simulink model "Parameter_estimation1"  (R2025b)
settings: Solver=VariableStepAuto  StartTime=0.0  StopTime=206057  FixedStep=1
libraries: fl_lib x15, nesl_utility x15, batt_lib x7, ee_lib x3
settings Model: Creator=faxio  LastModifiedBy=faxio

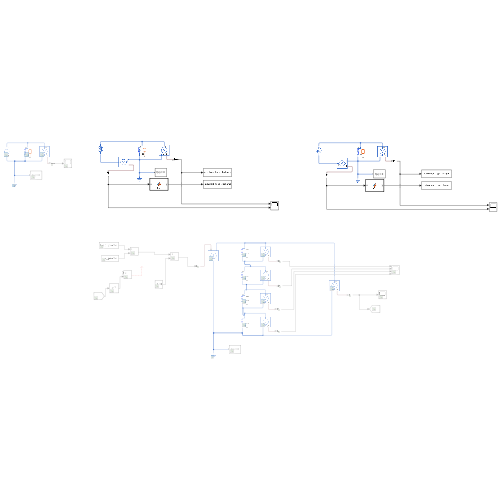
[thumbnail: Simulink's stored preview of the top-level diagram]
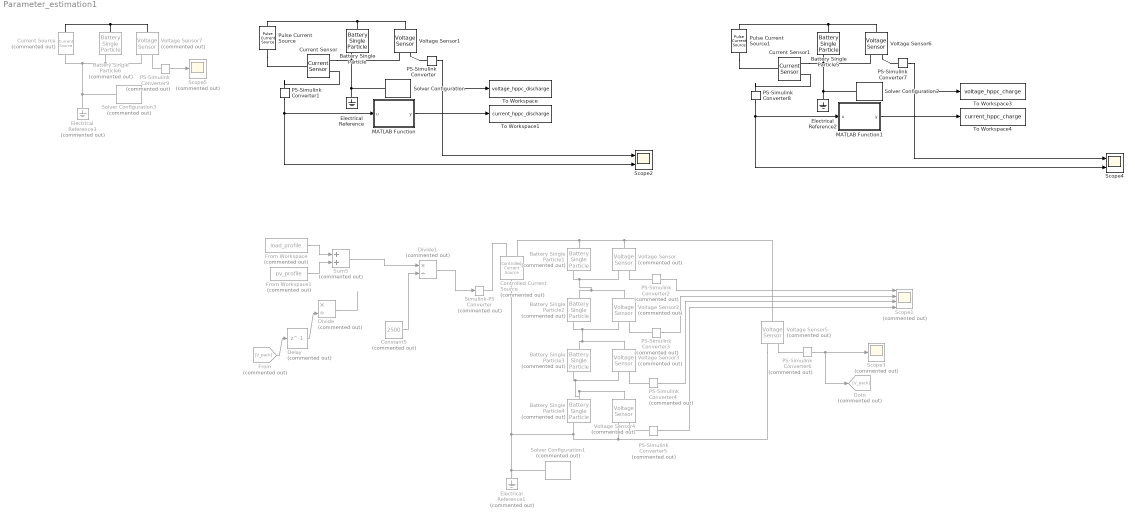
== system Parameter_estimation1 ==
  Battery Single Particle : batt_lib/Cells/Electrochemical/Battery Single Particle  ExtrapolationMethod=simscape.enum.extrapolation.nearest  ThicknessAnode=3.4E-5 m  ElectrolyteLayerCountAnode=10  ThicknessSeparator=2.5E-5 m  ElectrolyteLayerCountSeparator=5  ThicknessCathode=8E-5 m  ElectrolyteLayerCountCathode=10  ElectrodePlateArea=1.8E-1 m^2  ParticleRadiusAnode=5E-6 m  ShellCountAnode=10  ParticleRadiusCathode=5E-8 m  ShellCountCathode=10  ActiveMaterialVolumeFractionAnode=0.58  ActiveMaterialVolumeFractionCathode=0.374  StoichiometryBreakpointsSpecification=simscape.battery.enum.cells.electrochemical.StoichiometryBreakpointsSpecification.normalized  NormalizedStoichiometryBreakpoints=linspace(0.025, 0.975, 39)  OpenCircuitPotentialAnode=[.435; .325; .259; .221; .204; .194; .179; .166; .155; .145; .137; .131; .128; .127; .126; .125; .124; .123; .122; .121; .118; .117; .112; .109; .105; .1; .098; .095; .094; .093; .091; .09; .089; .088; .087; .086; .085; .084; .083] V  OpenCircuitPotentialCathode=[3.598; 3.53; 3.494; 3.474; 3.46; 3.455; 3.454; 3.453; 3.4528; 3.4526; 3.4524; 3.452; 3.4518; 3.4516; 3.4514; 3.4512; 3.451; 3.4508; 3.4506; 3.4503; 3.45; 3.4498; 3.4495; 3.4493; 3.449; 3.4488; 3.4486; 3.4484; 3.4482; 3.4479; 3.4477; 3.4475; 3.4473; 3.447; 3.4468; 3.4466; 3.4464; 3.4462; 3.4458] V  AbsoluteStoichiometryBreakpointsAnode=linspace(0.025, 0.975, 39)  OpenCircuitPotentialAbsoluteAnode=[.484; .335; .253; .209; .2; .181; .165; .151; .139; .131; .128; .125; .124; .124; .123; .122; .119; .117; .111; .108; .101; .098; .095; .093; .092; .088; .088; .088; .088; .087; .087; .087; .085; .082; .079; .071; .064; .049; .026] V  AbsoluteStoichiometryBreakpointsCathode=linspace(0.025, 0.975, 39)  OpenCircuitPotentialAbsoluteCathode=[3.81; 3.608; 3.512; 3.478; 3.459; 3.453; 3.45257; 3.45214; 3.45171; 3.45128; 3.45085; 3.45042; 3.44999; 3.44956; 3.44913; 3.4487; 3.44827; 3.44784; 3.44741; 3.44698; 3.44655; 3.44612; 3.44569; 3.44526; 3.44483; 3.4444; 3.44397; 3.44354; 3.44311; 3.44268; 3.44225; 3.44182; 3.44139; 3.44096; 3.44053; 3.44; 3.412; 3.304; 2.968] V  MaximumConcentrationAnode=30555 mol/m^3  MaximumStoichiometryAnode=0.811  MinimumStoichiometryAnode=0.0132  MaximumConcentrationCathode=22806 mol/m^3  MaximumStoichiometryCathode=0.74  MinimumStoichiometryCathode=0.035  ActiveMaterialDiffusionCoefficientAnode=3E-15 m^2/s  ActiveMaterialDiffusionCoefficientCathode=5.9E-20 m^2/s  ConductivityAnode=100 S/m  ConductivityCathode=0.5 S/m  CurrentCollectorResistance=0 Ohm  ElectrolyteVolumeFractionAnode=0.3874  ElectrolyteVolumeFractionSeparator=0.45  ElectrolyteVolumeFractionCathode=0.5725  ElectrolyteConductivity=0.29 S/m  BruggemanExponentAnode=1.5  BruggemanExponentSeparator=1.5  BruggemanExponentCathode=1.5  TransferenceNumber=0.363  ElectrolyteDiffusionCoefficient=2E-10 m^2/s  ChargeTransferRateAnode=8.8E-11 m^(5/2)/(mol^(1/2)*s)  ChargeTransferRateCathode=2.8E-13 m^(5/2)/(mol^(1/2)*s)  BatteryThermalMass=77 J/K  ArrheniusReferenceTemperature=298.15 K  ActiveMaterialDiffusionActivationEnergyAnode=39000 J/mol  ActiveMaterialDiffusionActivationEnergyCathode=35000 J/mol  ElectrolyteDiffusionActivationEnergy=26600 J/mol  ConductivityActivationEnergyAnode=3000 J/mol  ConductivityActivationEnergyCathode=3000 J/mol  ElectrolyteConductivityActivationEnergy=11000 J/mol  ChargeTransferActivationEnergyAnode=13000 J/mol  ChargeTransferActivationEnergyCathode=20000 J/mol  batteryCurrent_specify=off  batteryCurrent_priority=None  batteryCurrent=0 A  batteryCurrent_nominal_specify=off  batteryCurrent_nominal_value=1  batteryCurrent_nominal_unit=A  batteryVoltage_specify=off  batteryVoltage_priority=None  batteryVoltage=0 V  batteryVoltage_nominal_specify=off  batteryVoltage_nominal_value=1  batteryVoltage_nominal_unit=V  averageElectrolyteConcentration_specify=off  averageElectrolyteConcentration_priority=High  averageElectrolyteConcentration=1200 mol/m^3  averageElectrolyteConcentration_nominal_specify=off  averageElectrolyteConcentration_nominal_value=1  averageElectrolyteConcentration_nominal_unit=mol/m^3  stateOfCharge_specify=on  stateOfCharge_priority=High  stateOfCharge=1  stateOfCharge_nominal_specify=off  stateOfCharge_nominal_value=1  stateOfCharge_nominal_unit=1  batteryTemperature_specify=off  batteryTemperature_priority=High  batteryTemperature=298.15 K  batteryTemperature_nominal_specify=off  batteryTemperature_nominal_value=1  batteryTemperature_nominal_unit=K  power_dissipated_specify=off  power_dissipated_priority=None  power_dissipated=0 W  power_dissipated_nominal_specify=off  power_dissipated_nominal_value=1  power_dissipated_nominal_unit=W  heatGenerationRate_specify=off  heatGenerationRate_priority=None  heatGenerationRate=0 W  heatGenerationRate_nominal_specify=off  heatGenerationRate_nominal_value=1  heatGenerationRate_nominal_unit=W
      settings: InternalSimscapePortConfiguration="{\"Bottom\":[],\"Left\":[{\"id\":\"p\",\"label\":\"+\",\"type\":\"foundation.electrical.electrical\"}],\"Right\":[{\"id\":\"n\",\"label\":\"-\",\"type\":\"foundation.electrical.electrical\"},{\"id\":\"H\",\"label\":\"H\",\"type\":\"foundation.thermal.thermal\"}],\"Top\":[]}"
  Battery Single Particle{1..4,6} (5 alike) : batt_lib/Cells/Electrochemical/Battery Single Particle  Commented=on  ExtrapolationMethod=simscape.enum.extrapolation.nearest  ThicknessAnode=3.4E-5 m  ElectrolyteLayerCountAnode=10  ThicknessSeparator=2.5E-5 m  ElectrolyteLayerCountSeparator=5  ThicknessCathode=8E-5 m  ElectrolyteLayerCountCathode=10  ElectrodePlateArea=1.8E-1 m^2  ParticleRadiusAnode=5E-6 m  ShellCountAnode=10  ParticleRadiusCathode=5E-8 m  ShellCountCathode=10  ActiveMaterialVolumeFractionAnode=0.58  ActiveMaterialVolumeFractionCathode=0.374  StoichiometryBreakpointsSpecification=simscape.battery.enum.cells.electrochemical.StoichiometryBreakpointsSpecification.normalized  NormalizedStoichiometryBreakpoints=linspace(0.025, 0.975, 39)  OpenCircuitPotentialAnode=[.435; .325; .259; .221; .204; .194; .179; .166; .155; .145; .137; .131; .128; .127; .126; .125; .124; .123; .122; .121; .118; .117; .112; .109; .105; .1; .098; .095; .094; .093; .091; .09; .089; .088; .087; .086; .085; .084; .083] V  OpenCircuitPotentialCathode=[3.598; 3.53; 3.494; 3.474; 3.46; 3.455; 3.454; 3.453; 3.4528; 3.4526; 3.4524; 3.452; 3.4518; 3.4516; 3.4514; 3.4512; 3.451; 3.4508; 3.4506; 3.4503; 3.45; 3.4498; 3.4495; 3.4493; 3.449; 3.4488; 3.4486; 3.4484; 3.4482; 3.4479; 3.4477; 3.4475; 3.4473; 3.447; 3.4468; 3.4466; 3.4464; 3.4462; 3.4458] V  AbsoluteStoichiometryBreakpointsAnode=linspace(0.025, 0.975, 39)  OpenCircuitPotentialAbsoluteAnode=[.484; .335; .253; .209; .2; .181; .165; .151; .139; .131; .128; .125; .124; .124; .123; .122; .119; .117; .111; .108; .101; .098; .095; .093; .092; .088; .088; .088; .088; .087; .087; .087; .085; .082; .079; .071; .064; .049; .026] V  AbsoluteStoichiometryBreakpointsCathode=linspace(0.025, 0.975, 39)  OpenCircuitPotentialAbsoluteCathode=[3.81; 3.608; 3.512; 3.478; 3.459; 3.453; 3.45257; 3.45214; 3.45171; 3.45128; 3.45085; 3.45042; 3.44999; 3.44956; 3.44913; 3.4487; 3.44827; 3.44784; 3.44741; 3.44698; 3.44655; 3.44612; 3.44569; 3.44526; 3.44483; 3.4444; 3.44397; 3.44354; 3.44311; 3.44268; 3.44225; 3.44182; 3.44139; 3.44096; 3.44053; 3.44; 3.412; 3.304; 2.968] V  MaximumConcentrationAnode=30555 mol/m^3  MaximumStoichiometryAnode=0.811  MinimumStoichiometryAnode=0.0132  MaximumConcentrationCathode=22806 mol/m^3  MaximumStoichiometryCathode=0.74  MinimumStoichiometryCathode=0.035  ActiveMaterialDiffusionCoefficientAnode=3E-15 m^2/s  ActiveMaterialDiffusionCoefficientCathode=5.9E-20 m^2/s  ConductivityAnode=100 S/m  ConductivityCathode=0.5 S/m  CurrentCollectorResistance=0 Ohm  ElectrolyteVolumeFractionAnode=0.3874  ElectrolyteVolumeFractionSeparator=0.45  ElectrolyteVolumeFractionCathode=0.5725  ElectrolyteConductivity=0.29 S/m  BruggemanExponentAnode=1.5  BruggemanExponentSeparator=1.5  BruggemanExponentCathode=1.5  TransferenceNumber=0.363  ElectrolyteDiffusionCoefficient=2E-10 m^2/s  ChargeTransferRateAnode=8.8E-11 m^(5/2)/(mol^(1/2)*s)  ChargeTransferRateCathode=2.8E-13 m^(5/2)/(mol^(1/2)*s)  BatteryThermalMass=77 J/K  ArrheniusReferenceTemperature=298.15 K  ActiveMaterialDiffusionActivationEnergyAnode=39000 J/mol  ActiveMaterialDiffusionActivationEnergyCathode=35000 J/mol  ElectrolyteDiffusionActivationEnergy=26600 J/mol  ConductivityActivationEnergyAnode=3000 J/mol  ConductivityActivationEnergyCathode=3000 J/mol  ElectrolyteConductivityActivationEnergy=11000 J/mol  ChargeTransferActivationEnergyAnode=13000 J/mol  ChargeTransferActivationEnergyCathode=20000 J/mol  batteryCurrent_specify=off  batteryCurrent_priority=None  batteryCurrent=0 A  batteryCurrent_nominal_specify=off  batteryCurrent_nominal_value=1  batteryCurrent_nominal_unit=A  batteryVoltage_specify=off  batteryVoltage_priority=None  batteryVoltage=0 V  batteryVoltage_nominal_specify=off  batteryVoltage_nominal_value=1  batteryVoltage_nominal_unit=V  averageElectrolyteConcentration_specify=off  averageElectrolyteConcentration_priority=High  averageElectrolyteConcentration=1200 mol/m^3  averageElectrolyteConcentration_nominal_specify=off  averageElectrolyteConcentration_nominal_value=1  averageElectrolyteConcentration_nominal_unit=mol/m^3  stateOfCharge_specify=on  stateOfCharge_priority=High  stateOfCharge=1  stateOfCharge_nominal_specify=off  stateOfCharge_nominal_value=1  stateOfCharge_nominal_unit=1  batteryTemperature_specify=off  batteryTemperature_priority=High  batteryTemperature=298.15 K  batteryTemperature_nominal_specify=off  batteryTemperature_nominal_value=1  batteryTemperature_nominal_unit=K  power_dissipated_specify=off  power_dissipated_priority=None  power_dissipated=0 W  power_dissipated_nominal_specify=off  power_dissipated_nominal_value=1  power_dissipated_nominal_unit=W  heatGenerationRate_specify=off  heatGenerationRate_priority=None  heatGenerationRate=0 W  heatGenerationRate_nominal_specify=off  heatGenerationRate_nominal_value=1  heatGenerationRate_nominal_unit=W
      settings: InternalSimscapePortConfiguration="{\"Bottom\":[],\"Left\":[{\"id\":\"p\",\"label\":\"+\",\"type\":\"foundation.electrical.electrical\"}],\"Right\":[{\"id\":\"n\",\"label\":\"-\",\"type\":\"foundation.electrical.electrical\"},{\"id\":\"H\",\"label\":\"H\",\"type\":\"foundation.thermal.thermal\"}],\"Top\":[]}"
  Battery Single Particle5 : batt_lib/Cells/Electrochemical/Battery Single Particle  ExtrapolationMethod=simscape.enum.extrapolation.nearest  ThicknessAnode=3.4E-5 m  ElectrolyteLayerCountAnode=10  ThicknessSeparator=2.5E-5 m  ElectrolyteLayerCountSeparator=5  ThicknessCathode=8E-5 m  ElectrolyteLayerCountCathode=10  ElectrodePlateArea=1.8E-1 m^2  ParticleRadiusAnode=5E-6 m  ShellCountAnode=10  ParticleRadiusCathode=5E-8 m  ShellCountCathode=10  ActiveMaterialVolumeFractionAnode=0.58  ActiveMaterialVolumeFractionCathode=0.374  StoichiometryBreakpointsSpecification=simscape.battery.enum.cells.electrochemical.StoichiometryBreakpointsSpecification.normalized  NormalizedStoichiometryBreakpoints=linspace(0.025, 0.975, 39)  OpenCircuitPotentialAnode=[.435; .325; .259; .221; .204; .194; .179; .166; .155; .145; .137; .131; .128; .127; .126; .125; .124; .123; .122; .121; .118; .117; .112; .109; .105; .1; .098; .095; .094; .093; .091; .09; .089; .088; .087; .086; .085; .084; .083] V  OpenCircuitPotentialCathode=[3.598; 3.53; 3.494; 3.474; 3.46; 3.455; 3.454; 3.453; 3.4528; 3.4526; 3.4524; 3.452; 3.4518; 3.4516; 3.4514; 3.4512; 3.451; 3.4508; 3.4506; 3.4503; 3.45; 3.4498; 3.4495; 3.4493; 3.449; 3.4488; 3.4486; 3.4484; 3.4482; 3.4479; 3.4477; 3.4475; 3.4473; 3.447; 3.4468; 3.4466; 3.4464; 3.4462; 3.4458] V  AbsoluteStoichiometryBreakpointsAnode=linspace(0.025, 0.975, 39)  OpenCircuitPotentialAbsoluteAnode=[.484; .335; .253; .209; .2; .181; .165; .151; .139; .131; .128; .125; .124; .124; .123; .122; .119; .117; .111; .108; .101; .098; .095; .093; .092; .088; .088; .088; .088; .087; .087; .087; .085; .082; .079; .071; .064; .049; .026] V  AbsoluteStoichiometryBreakpointsCathode=linspace(0.025, 0.975, 39)  OpenCircuitPotentialAbsoluteCathode=[3.81; 3.608; 3.512; 3.478; 3.459; 3.453; 3.45257; 3.45214; 3.45171; 3.45128; 3.45085; 3.45042; 3.44999; 3.44956; 3.44913; 3.4487; 3.44827; 3.44784; 3.44741; 3.44698; 3.44655; 3.44612; 3.44569; 3.44526; 3.44483; 3.4444; 3.44397; 3.44354; 3.44311; 3.44268; 3.44225; 3.44182; 3.44139; 3.44096; 3.44053; 3.44; 3.412; 3.304; 2.968] V  MaximumConcentrationAnode=30555 mol/m^3  MaximumStoichiometryAnode=0.811  MinimumStoichiometryAnode=0.0132  MaximumConcentrationCathode=22806 mol/m^3  MaximumStoichiometryCathode=0.74  MinimumStoichiometryCathode=0.035  ActiveMaterialDiffusionCoefficientAnode=3E-15 m^2/s  ActiveMaterialDiffusionCoefficientCathode=5.9E-20 m^2/s  ConductivityAnode=100 S/m  ConductivityCathode=0.5 S/m  CurrentCollectorResistance=0 Ohm  ElectrolyteVolumeFractionAnode=0.3874  ElectrolyteVolumeFractionSeparator=0.45  ElectrolyteVolumeFractionCathode=0.5725  ElectrolyteConductivity=0.29 S/m  BruggemanExponentAnode=1.5  BruggemanExponentSeparator=1.5  BruggemanExponentCathode=1.5  TransferenceNumber=0.363  ElectrolyteDiffusionCoefficient=2E-10 m^2/s  ChargeTransferRateAnode=8.8E-11 m^(5/2)/(mol^(1/2)*s)  ChargeTransferRateCathode=2.8E-13 m^(5/2)/(mol^(1/2)*s)  BatteryThermalMass=77 J/K  ArrheniusReferenceTemperature=298.15 K  ActiveMaterialDiffusionActivationEnergyAnode=39000 J/mol  ActiveMaterialDiffusionActivationEnergyCathode=35000 J/mol  ElectrolyteDiffusionActivationEnergy=26600 J/mol  ConductivityActivationEnergyAnode=3000 J/mol  ConductivityActivationEnergyCathode=3000 J/mol  ElectrolyteConductivityActivationEnergy=11000 J/mol  ChargeTransferActivationEnergyAnode=13000 J/mol  ChargeTransferActivationEnergyCathode=20000 J/mol  batteryCurrent_specify=off  batteryCurrent_priority=None  batteryCurrent=0 A  batteryCurrent_nominal_specify=off  batteryCurrent_nominal_value=1  batteryCurrent_nominal_unit=A  batteryVoltage_specify=off  batteryVoltage_priority=None  batteryVoltage=0 V  batteryVoltage_nominal_specify=off  batteryVoltage_nominal_value=1  batteryVoltage_nominal_unit=V  averageElectrolyteConcentration_specify=off  averageElectrolyteConcentration_priority=High  averageElectrolyteConcentration=1200 mol/m^3  averageElectrolyteConcentration_nominal_specify=off  averageElectrolyteConcentration_nominal_value=1  averageElectrolyteConcentration_nominal_unit=mol/m^3  stateOfCharge_specify=on  stateOfCharge_priority=High  stateOfCharge=0  stateOfCharge_nominal_specify=off  stateOfCharge_nominal_value=1  stateOfCharge_nominal_unit=1  batteryTemperature_specify=off  batteryTemperature_priority=High  batteryTemperature=298.15 K  batteryTemperature_nominal_specify=off  batteryTemperature_nominal_value=1  batteryTemperature_nominal_unit=K  power_dissipated_specify=off  power_dissipated_priority=None  power_dissipated=0 W  power_dissipated_nominal_specify=off  power_dissipated_nominal_value=1  power_dissipated_nominal_unit=W  heatGenerationRate_specify=off  heatGenerationRate_priority=None  heatGenerationRate=0 W  heatGenerationRate_nominal_specify=off  heatGenerationRate_nominal_value=1  heatGenerationRate_nominal_unit=W
      settings: InternalSimscapePortConfiguration="{\"Bottom\":[],\"Left\":[{\"id\":\"p\",\"label\":\"+\",\"type\":\"foundation.electrical.electrical\"}],\"Right\":[{\"id\":\"n\",\"label\":\"-\",\"type\":\"foundation.electrical.electrical\"},{\"id\":\"H\",\"label\":\"H\",\"type\":\"foundation.thermal.thermal\"}],\"Top\":[]}"
  Constant5 : Constant  Commented=on  Value=2500
  Controlled Current Source : fl_lib/Electrical/Electrical Sources/Controlled Current Source  Commented=on
  Current Sensor : fl_lib/Electrical/Electrical Sensors/Current Sensor
  Current Sensor1 : fl_lib/Electrical/Electrical Sensors/Current Sensor
  Current Source : ee_lib/Sources/Current Source  Commented=on  dc_current=1 A  ac_current=0 A  ac_shift=0 rad  ac_frequency=60 Hz  noise_mode=ee.enum.sources.noise.Disabled  PSD=0 A^2/Hz  sample_time=1e-3 s  repeatability=ee.enum.sources.repeatability.NotRepeatable  user_seed=0  auto_seed=545404223  i_specify=off  i_priority=None  i=0 A  i_nominal_specify=off  i_nominal_value=1  i_nominal_unit=A  v_specify=off  v_priority=None  v=0 V  v_nominal_specify=off  v_nominal_value=1  v_nominal_unit=V
  Delay : Delay  Commented=on  DelayLength=1  InputProcessing=Columns as channels (frame based)
  Divide : Product  Commented=on  Inputs=*/
  Divide1 : Product  Commented=on  Inputs=*/
  Electrical Reference : fl_lib/Electrical/Electrical Elements/Electrical Reference
  Electrical Reference1 : fl_lib/Electrical/Electrical Elements/Electrical Reference  Commented=on
  Electrical Reference2 : fl_lib/Electrical/Electrical Elements/Electrical Reference
  Electrical Reference3 : fl_lib/Electrical/Electrical Elements/Electrical Reference  Commented=on
  From : From  Commented=on  GotoTag=V_pack
  From Workspace : FromWorkspace  Commented=on  VariableName=load_profile
  From Workspace1 : FromWorkspace  Commented=on  VariableName=pv_profile
  Goto : Goto  Commented=on  GotoTag=V_pack
  MATLAB Function : MATLAB Function  TreatAsAtomicUnit=on
  MATLAB Function1 : MATLAB Function  TreatAsAtomicUnit=on
  PS-Simulink Converter{,1,7..8} (4 alike) : nesl_utility/PS-Simulink Converter  PhysicalDomain=network_engine_domain  SubClassName=ps_output  LeftPortType=input  RightPortType=output  PseudoPeriodic=off  Frequencies=[]  VectorFormat=inherit  Unit=inherit  AffineConversion=off
  PS-Simulink Converter{2..6,9} (6 alike) : nesl_utility/PS-Simulink Converter  Commented=on  PhysicalDomain=network_engine_domain  SubClassName=ps_output  LeftPortType=input  RightPortType=output  PseudoPeriodic=off  Frequencies=[]  VectorFormat=inherit  Unit=inherit  AffineConversion=off
  Pulse Current Source : ee_lib/Additional Components/SPICE Sources/Pulse Current Source  I1=0 A  I2=1 A  TD=0 s  TR=1e-9 s  TF=1e-9 s  PW=80 s  PER=2000 s  Gmin_param=ee.enum.gminParam.yes
      settings: LibrarySourceBlock=ee_lib/Sources/Pulse Current Source  InternalSimscapePortConfiguration="{\"Bottom\":[],\"Left\":[{\"id\":\"p\",\"label\":\"\",\"type\":\"foundation.electrical.electrical\"}],\"Right\":[{\"id\":\"n\",\"label\":\"\",\"type\":\"foundation.electrical.electrical\"}],\"Top\":[]}"
  Pulse Current Source1 : ee_lib/Additional Components/SPICE Sources/Pulse Current Source  I1=0 A  I2=-1 A  TD=0 s  TR=1e-9 s  TF=1e-9 s  PW=80 s  PER=2000 s  Gmin_param=ee.enum.gminParam.yes
      settings: LibrarySourceBlock=ee_lib/Sources/Pulse Current Source  InternalSimscapePortConfiguration="{\"Bottom\":[],\"Left\":[{\"id\":\"p\",\"label\":\"\",\"type\":\"foundation.electrical.electrical\"}],\"Right\":[{\"id\":\"n\",\"label\":\"\",\"type\":\"foundation.electrical.electrical\"}],\"Top\":[]}"
  Scope1 : Scope  Commented=on  NumInputPorts=4
      settings: ActiveDisplayYMinimum=-1  ActiveDisplayYMaximum=1
  Scope2 : Scope  NumInputPorts=2
      settings: ActiveDisplayYMinimum=2.8332357800564645  ActiveDisplayYMaximum=3.5907515817104656  DataLoggingVariableName=ScopeData2
  Scope3 : Scope  Commented=on
      settings: ActiveDisplayYMinimum=11.851885488512112  ActiveDisplayYMaximum=13.610571697723437  DataLoggingVariableName=ScopeData3
  Scope4 : Scope  NumInputPorts=2
      settings: ActiveDisplayYMinimum=2.9421106052239043  ActiveDisplayYMaximum=3.6290045529629764
  Scope5 : Scope  Commented=on
      settings: ActiveDisplayYMinimum=2.8486897054184919  ActiveDisplayYMaximum=3.5597839817126782  DataLoggingVariableName=ScopeData4
  Simulink-PS Converter : nesl_utility/Simulink-PS Converter  Commented=on  PhysicalDomain=network_engine_domain  SubClassName=ps_input  LeftPortType=input  RightPortType=output  PseudoPeriodic=off  Frequencies=[]  NoiseDistribution=none  NoiseParameters=[]  Unit=1  AffineConversion=off  FilteringAndDerivatives=provide  SimscapeFilterOrder=1  InputFilterTimeConstant=0.001  UdotUserProvided=0
  Solver Configuration : nesl_utility/Solver Configuration  PhysicalDomain=network_engine_domain  SubClassName=solver  LeftPortType=input  RightPortType=generic  Tones=[]  Harmonics=[]  SimulateNoise=off  Profile=off  UseLocalSampling=off  EnableSwitchedLinearOptims=on  FrequencyDomain=off  UseCCode=off  RelTol=0.001  AbsTol=0.001  MinStep=1e-09  ToWorkspace=off  RevertToSquareIcSolve=off  NumHomotopyIterations=100  PhasorMode=off  PhasorModeNumHarmonics=1  ConsistencySolver=NEWTON_XTOL_AFTER_FTOL  IndexReductionMethod=DerivativeReplacement  DoDC=off  ResidualTolerance=1e-09  ConsistencyTolSource=GLOBAL  ConsistencyAbsTol=0.001  ConsistencyRelTol=0.001  ConsistencyTolFactor=0.001  UseLocalSolver=off  LocalSolverChoice=NE_BACKWARD_EULER_ADVANCER  ResolveIndetEquations=on  FunctionEvalNumThread=1  LocalSolverSampleTime=0.001  DoFixedCost=off  MaxNonlinIter=3  MaxModeIter=2  ComputeImpulses=off  ImpulseIterations=2  LinearAlgebra=auto  LinearAlgebraNumThread=0  EquationFormulation=NE_TIME_EF  DelaysMemoryBudget=1024  AutomaticFiltering=on  FilteringTimeConstant=0.001  PartitionStorageMethod=AS_NEEDED  PartitionMemoryBudget=1024  PartitionMethod=ROBUST  MultibodyUseLocalSolver=off  MultibodyLocalSolverChoice=ODE1  MultibodyLocalSolverSampleTime=0.001
  Solver Configuration1 : nesl_utility/Solver Configuration  Commented=on  PhysicalDomain=network_engine_domain  SubClassName=solver  LeftPortType=input  RightPortType=generic  Tones=[]  Harmonics=[]  SimulateNoise=off  Profile=off  UseLocalSampling=off  EnableSwitchedLinearOptims=on  FrequencyDomain=off  UseCCode=off  RelTol=0.001  AbsTol=0.001  MinStep=1e-09  ToWorkspace=off  RevertToSquareIcSolve=off  NumHomotopyIterations=100  PhasorMode=off  PhasorModeNumHarmonics=1  ConsistencySolver=NEWTON_XTOL_AFTER_FTOL  IndexReductionMethod=DerivativeReplacement  DoDC=off  ResidualTolerance=1e-09  ConsistencyTolSource=GLOBAL  ConsistencyAbsTol=0.001  ConsistencyRelTol=0.001  ConsistencyTolFactor=0.001  UseLocalSolver=off  LocalSolverChoice=NE_BACKWARD_EULER_ADVANCER  ResolveIndetEquations=on  FunctionEvalNumThread=1  LocalSolverSampleTime=0.001  DoFixedCost=off  MaxNonlinIter=3  MaxModeIter=2  ComputeImpulses=off  ImpulseIterations=2  LinearAlgebra=auto  LinearAlgebraNumThread=0  EquationFormulation=NE_TIME_EF  DelaysMemoryBudget=1024  AutomaticFiltering=on  FilteringTimeConstant=0.001  PartitionStorageMethod=AS_NEEDED  PartitionMemoryBudget=1024  PartitionMethod=ROBUST  MultibodyUseLocalSolver=off  MultibodyLocalSolverChoice=ODE1  MultibodyLocalSolverSampleTime=0.001
  Solver Configuration2 : nesl_utility/Solver Configuration  PhysicalDomain=network_engine_domain  SubClassName=solver  LeftPortType=input  RightPortType=generic  Tones=[]  Harmonics=[]  SimulateNoise=off  Profile=off  UseLocalSampling=off  EnableSwitchedLinearOptims=on  FrequencyDomain=off  UseCCode=off  RelTol=0.001  AbsTol=0.001  MinStep=1e-09  ToWorkspace=off  RevertToSquareIcSolve=off  NumHomotopyIterations=100  PhasorMode=off  PhasorModeNumHarmonics=1  ConsistencySolver=NEWTON_XTOL_AFTER_FTOL  IndexReductionMethod=DerivativeReplacement  DoDC=off  ResidualTolerance=1e-09  ConsistencyTolSource=GLOBAL  ConsistencyAbsTol=0.001  ConsistencyRelTol=0.001  ConsistencyTolFactor=0.001  UseLocalSolver=off  LocalSolverChoice=NE_BACKWARD_EULER_ADVANCER  ResolveIndetEquations=on  FunctionEvalNumThread=1  LocalSolverSampleTime=0.001  DoFixedCost=off  MaxNonlinIter=3  MaxModeIter=2  ComputeImpulses=off  ImpulseIterations=2  LinearAlgebra=auto  LinearAlgebraNumThread=0  EquationFormulation=NE_TIME_EF  DelaysMemoryBudget=1024  AutomaticFiltering=on  FilteringTimeConstant=0.001  PartitionStorageMethod=AS_NEEDED  PartitionMemoryBudget=1024  PartitionMethod=ROBUST  MultibodyUseLocalSolver=off  MultibodyLocalSolverChoice=ODE1  MultibodyLocalSolverSampleTime=0.001
  Solver Configuration3 : nesl_utility/Solver Configuration  Commented=on  PhysicalDomain=network_engine_domain  SubClassName=solver  LeftPortType=input  RightPortType=generic  Tones=[]  Harmonics=[]  SimulateNoise=off  Profile=off  UseLocalSampling=off  EnableSwitchedLinearOptims=on  FrequencyDomain=off  UseCCode=off  RelTol=0.001  AbsTol=0.001  MinStep=1e-09  ToWorkspace=off  RevertToSquareIcSolve=off  NumHomotopyIterations=100  PhasorMode=off  PhasorModeNumHarmonics=1  ConsistencySolver=NEWTON_XTOL_AFTER_FTOL  IndexReductionMethod=DerivativeReplacement  DoDC=off  ResidualTolerance=1e-09  ConsistencyTolSource=GLOBAL  ConsistencyAbsTol=0.001  ConsistencyRelTol=0.001  ConsistencyTolFactor=0.001  UseLocalSolver=off  LocalSolverChoice=NE_BACKWARD_EULER_ADVANCER  ResolveIndetEquations=on  FunctionEvalNumThread=1  LocalSolverSampleTime=0.001  DoFixedCost=off  MaxNonlinIter=3  MaxModeIter=2  ComputeImpulses=off  ImpulseIterations=2  LinearAlgebra=auto  LinearAlgebraNumThread=0  EquationFormulation=NE_TIME_EF  DelaysMemoryBudget=1024  AutomaticFiltering=on  FilteringTimeConstant=0.001  PartitionStorageMethod=AS_NEEDED  PartitionMemoryBudget=1024  PartitionMethod=ROBUST  MultibodyUseLocalSolver=off  MultibodyLocalSolverChoice=ODE1  MultibodyLocalSolverSampleTime=0.001
  Sum5 : Sum  Commented=on
  To Workspace : ToWorkspace  VariableName=voltage_hppc_discharge  SaveFormat=Timeseries  SampleTime=1
  To Workspace1 : ToWorkspace  VariableName=current_hppc_discharge  SaveFormat=Timeseries  SampleTime=1
  To Workspace3 : ToWorkspace  VariableName=voltage_hppc_charge  SaveFormat=Timeseries  SampleTime=1
  To Workspace4 : ToWorkspace  VariableName=current_hppc_charge  SaveFormat=Timeseries  SampleTime=1
  Voltage Sensor{,2..5,7} (6 alike) : fl_lib/Electrical/Electrical Sensors/Voltage Sensor  Commented=on
  Voltage Sensor1 : fl_lib/Electrical/Electrical Sensors/Voltage Sensor
  Voltage Sensor6 : fl_lib/Electrical/Electrical Sensors/Voltage Sensor
  wires:
  Divide1/1 -> Simulink-PS Converter/1
  Constant5/1 -> Divide1/2
  From Workspace/1 -> Sum5/1
  From Workspace1/1 -> Sum5/2
  PS-Simulink Converter/1 -> Scope2/1, To Workspace/1
  PS-Simulink Converter2/1 -> Scope1/1
  PS-Simulink Converter3/1 -> Scope1/2
  PS-Simulink Converter4/1 -> Scope1/3
  PS-Simulink Converter5/1 -> Scope1/4
  PS-Simulink Converter6/1 -> Goto/1, Scope3/1
  From/1 -> Delay/1
  Delay/1 -> Divide/2
  Sum5/1 -> Divide1/1
  Divide/1 -> ?
  PS-Simulink Converter1/1 -> MATLAB Function/1(u), Scope2/2
  PS-Simulink Converter8/1 -> MATLAB Function1/1(u), Scope4/2
  PS-Simulink Converter7/1 -> Scope4/1, To Workspace3/1
  MATLAB Function1/1(y) -> To Workspace4/1
  PS-Simulink Converter9/1 -> Scope5/1
  MATLAB Function/1(y) -> To Workspace1/1
  connections:
  Battery Single Particle/LConn1 -- Pulse Current Source/LConn1 -- Voltage Sensor1/LConn1
  Battery Single Particle/RConn1 -- Electrical Reference/LConn1 -- Solver Configuration/RConn1 -- Current Sensor/RConn2 -- Voltage Sensor1/RConn2
  Battery Single Particle2/LConn1 -- Battery Single Particle1/RConn1 -- Voltage Sensor/RConn2 -- Voltage Sensor2/LConn1
  Battery Single Particle1/LConn1 -- Controlled Current Source/RConn2 -- Voltage Sensor5/LConn1 -- Voltage Sensor/LConn1
  Simulink-PS Converter/RConn1 -- Controlled Current Source/RConn1
  PS-Simulink Converter/LConn1 -- Voltage Sensor1/RConn1
  PS-Simulink Converter1/LConn1 -- Current Sensor/RConn1
  Pulse Current Source/RConn1 -- Current Sensor/LConn1
  Solver Configuration1/RConn1 -- Controlled Current Source/LConn1 -- Voltage Sensor4/RConn2 -- Voltage Sensor5/RConn2 -- Battery Single Particle4/RConn1 -- Electrical Reference1/LConn1
  Voltage Sensor3/RConn2 -- Voltage Sensor4/LConn1 -- Battery Single Particle4/LConn1 -- Battery Single Particle3/RConn1
  Voltage Sensor2/RConn2 -- Voltage Sensor3/LConn1 -- Battery Single Particle3/LConn1 -- Battery Single Particle2/RConn1
  Voltage Sensor/RConn1 -- PS-Simulink Converter2/LConn1
  Voltage Sensor2/RConn1 -- PS-Simulink Converter3/LConn1
  Voltage Sensor3/RConn1 -- PS-Simulink Converter4/LConn1
  Voltage Sensor4/RConn1 -- PS-Simulink Converter5/LConn1
  Voltage Sensor5/RConn1 -- PS-Simulink Converter6/LConn1
  Voltage Sensor6/RConn2 -- Battery Single Particle5/RConn1 -- Electrical Reference2/LConn1 -- Solver Configuration2/RConn1 -- Current Sensor1/RConn2
  Voltage Sensor6/LConn1 -- Battery Single Particle5/LConn1 -- Pulse Current Source1/LConn1
  Pulse Current Source1/RConn1 -- Current Sensor1/LConn1
  PS-Simulink Converter8/LConn1 -- Current Sensor1/RConn1
  PS-Simulink Converter7/LConn1 -- Voltage Sensor6/RConn1
  Solver Configuration3/RConn1 -- Electrical Reference3/LConn1 -- Current Source/LConn1 -- Voltage Sensor7/RConn2 -- Battery Single Particle6/RConn1
  Battery Single Particle6/LConn1 -- Current Source/RConn1 -- Voltage Sensor7/LConn1
  PS-Simulink Converter9/LConn1 -- Voltage Sensor7/RConn1

== matlab function Parameter_estimation1/MATLAB Function ==
  data: u input; y output
function y = fcn(u)

if u<= 0.001
    y=0;
else
    y=u;
end

== matlab function Parameter_estimation1/MATLAB Function1 ==
  data: u input; y output
function y = fcn(u)
if u>= -0.001
    y=0;
else
    y=u;
end
